simulink model "ZEH_PV_grid"  (R2020a)
settings: Solver=VariableStepAuto  StartTime=0.0  StopTime=24*60*60  RelTol=1e-3
InitFcn:
  | SENSE2_dat
values from neighbouring files (symbols this model uses):
  apv = [72 76 288 252 0 0 40 360 460 168 84]  *1E2    [ZEH_dat_summer.m]    (also in ZEH_dat_winter.m)
  cab = [0.206 0.29 0.36 285 335 ... (first row only)    [ZEH_dat_summer.m]    (also in ZEH_dat_winter.m)
  cons = [0.64,0.60,0.58,0.56,0.56,0.58,0.64,0.76,0.87,0.95,0.99,1.00,0.99,1.00,1.00,0.97,0.96,0.96,0.93,0.92,0.92,0.93,0.87,0.72]    [ZEH_dat_summer.m]    (also in ZEH_dat_winter.m = [0.67,0.63,0.60,0.59,0.59,0.60,0.74,0.86,0.85,0.96,0.96,0.95)
  inic = 0.00095    [ZEH_dat_summer.m]    (also in ZEH_dat_winter.m)
  irr = [0,0,0,0,0,0,0,0,0,0,0,0,0,0,0,0,0,0,0,0,0,0,0,0,0,0,0,0,0,0,0,0,0,0,0,0,0,0,0,0,0,0,0,0,0,0,0,0,0,0,0,0,0,0,0,0,0,0,0,0,0,0,0,0,0,0,0,0,0,0,0,0,0,0,0,0,0,0,0,0,0,0,0,0,0,0,0,0,0,0,0,0,0,0,0,0,0,0,0,0,0,0,0,0,0,0,0,0,0,0,0,0,0,0,0,0,0,0,0,0,0,0,0,0,0,0,0,0,0,0,0,0,0,0,0,0,0,0,0,0,0,0,0,0,0,0,0,0,0,0,0,0,0,0,0,0,0,0,0,0,0,0,0,0,0,0,0,0,0,0,0,0,0,0,0,0,0,0,0,0,0,0,0,0,0,0,0,0,0,0,0,0,0,0,0,0,0,0,0,0 ...(+12851 chars)    [ZEH_dat_summer.m]    (also in ZEH_dat_winter.m = zeros(1,length(irr)))
  lp = 0.002    [ZEH_dat_summer.m]    (also in ZEH_dat_winter.m)
  SL = [7.57 8.06 30.73 53.01 133.26 219.22 4.00 37.53 48.38 17.80 9.04]*1E-3    [ZEH_dat_summer.m]    (also in ZEH_dat_winter.m)
  time = [1,1.01666666666667,1.03333333333333,1.05000000000000,1.06666666666667,1.08333333333333,1.10000000000000,1.11666666666667,1.13333333333333,1.15000000000000,1.16666666666667,1.18333333333333,1.20000000000000,1.21666666666667,1.23333333333333,1.25000000000000,1.26666666666667,1.28333333333333,1.30000000000000,1.31666666666667,1.33333333333333,1.35000000000000,1.36666666666667,1.38333333333333,1.4000 ...(+22733 chars)    [ZEH_dat_summer.m]    (also in ZEH_dat_winter.m)
  to = 0.1    [ZEH_dat_summer.m]    (also in ZEH_dat_winter.m)
undefined symbols (not defined in the file or in its folder): A, B, C, D1, Dd, Delta, j
libraries: powerlib x166, simulink_extras x12, powerlib_meascontrol x11, simulink x2, factslib x2
(part 1 of 5)
settings Model: Creator=nitbh  LastModifiedBy=nitbh

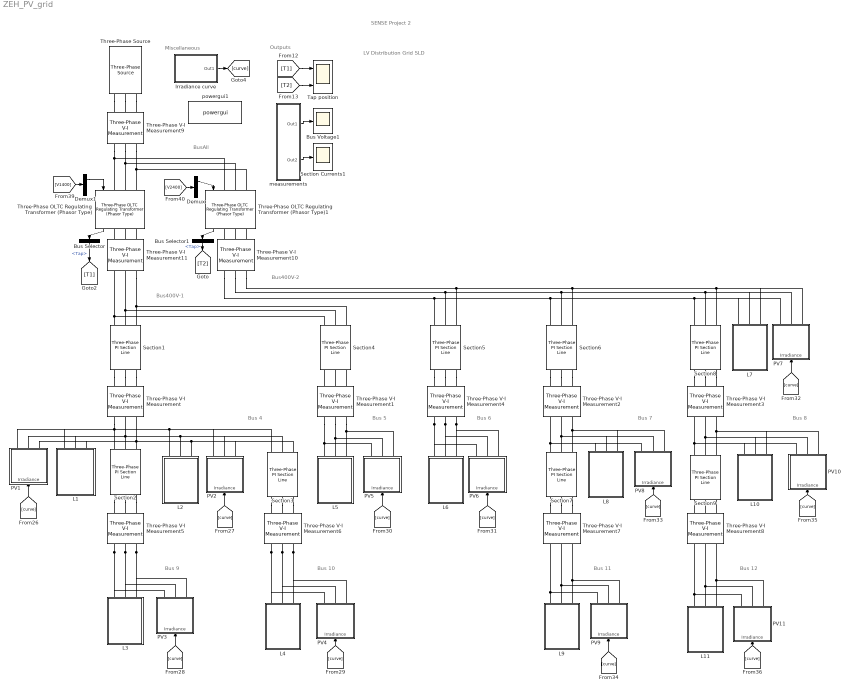
== system ZEH_PV_grid ==
  note: SENSE Project 2
  note: LV Distribution Grid SLD
  note: Outputs
  note: Miscellaneous
  note: Bus 4
  note: Bus 5
  note: Bus 9
  note: Bus 10
  note: Bus 11
  note: Bus 6
  note: Bus 7
  note: Bus 8
  note: Bus 12
  note: Bus400V-1
  note: Bus400V-2
  note: BusAll
  " Irradiance curve" : Subsystem
  Bus Selector : BusSelector  OutputSignals=Tap
  Bus Selector1 : BusSelector  OutputSignals=Tap
  Bus Voltage1 : Scope
  Demux : Demux  Outputs=3
  Demux1 : Demux  Outputs=3
  L1 : Subsystem  mask{nomPower=SL(1), PF=0.95, timestep=60, datas=cons}
      mask prompts: nomPower "Nominal Power (MW)"; PF "Power factor"; timestep "Timestep (minutes)"; datas "Consumption datas"
      mask DialogControl DescGroupVar Prompt: Load profile
      mask DialogControl DescTextVar Prompt: The load profile allows you to fix a nominal power and and a power factor. It is also needed to specify the timestep used for the consumption datas. Finally, a vector expresses the consumption profile. It has to be expressed in per unit. It is imperative that the length of the vector fits with the timestep used.
      mask Display: image(imread('Residential.jpg'))
  L10 : Subsystem  mask{nomPower=SL(10), PF=0.95, timestep=60, datas=cons}
      mask prompts: nomPower "Nominal Power (MW)"; PF "Power factor"; timestep "Timestep (minutes)"; datas "Consumption datas"
      mask DialogControl DescGroupVar Prompt: Load profile
      mask DialogControl DescTextVar Prompt: The load profile allows you to fix a nominal power and and a power factor. It is also needed to specify the timestep used for the consumption datas. Finally, a vector expresses the consumption profile. It has to be expressed in per unit. It is imperative that the length of the vector fits with the timestep used.
      mask Display: image(imread('Residential.jpg'))
  L11 : Subsystem  mask{nomPower=SL(11), PF=0.95, timestep=60, datas=cons}
      mask prompts: nomPower "Nominal Power (MW)"; PF "Power factor"; timestep "Timestep (minutes)"; datas "Consumption datas"
      mask DialogControl DescGroupVar Prompt: Load profile
      mask DialogControl DescTextVar Prompt: The load profile allows you to fix a nominal power and and a power factor. It is also needed to specify the timestep used for the consumption datas. Finally, a vector expresses the consumption profile. It has to be expressed in per unit. It is imperative that the length of the vector fits with the timestep used.
      mask Display: image(imread('Residential.jpg'))
  L2 : Subsystem  mask{nomPower=SL(2), PF=0.95, timestep=60, datas=cons}
      mask prompts: nomPower "Nominal Power (MW)"; PF "Power factor"; timestep "Timestep (minutes)"; datas "Consumption datas"
      mask DialogControl DescGroupVar Prompt: Load profile
      mask DialogControl DescTextVar Prompt: The load profile allows you to fix a nominal power and and a power factor. It is also needed to specify the timestep used for the consumption datas. Finally, a vector expresses the consumption profile. It has to be expressed in per unit. It is imperative that the length of the vector fits with the timestep used.
      mask Display: image(imread('Residential.jpg'))
  L3 : Subsystem  mask{nomPower=SL(3), PF=0.95, timestep=60, datas=cons}
      mask prompts: nomPower "Nominal Power (MW)"; PF "Power factor"; timestep "Timestep (minutes)"; datas "Consumption datas"
      mask DialogControl DescGroupVar Prompt: Load profile
      mask DialogControl DescTextVar Prompt: The load profile allows you to fix a nominal power and and a power factor. It is also needed to specify the timestep used for the consumption datas. Finally, a vector expresses the consumption profile. It has to be expressed in per unit. It is imperative that the length of the vector fits with the timestep used.
      mask Display: image(imread('Residential.jpg'))
  L4 : Subsystem  mask{nomPower=SL(4), PF=0.95, timestep=60, datas=cons}
      mask prompts: nomPower "Nominal Power (MW)"; PF "Power factor"; timestep "Timestep (minutes)"; datas "Consumption datas"
      mask DialogControl DescGroupVar Prompt: Load profile
      mask DialogControl DescTextVar Prompt: The load profile allows you to fix a nominal power and and a power factor. It is also needed to specify the timestep used for the consumption datas. Finally, a vector expresses the consumption profile. It has to be expressed in per unit. It is imperative that the length of the vector fits with the timestep used.
      mask Display: image(imread('Residential.jpg'))
  L5 : Subsystem  mask{nomPower=SL(5), PF=0.95, timestep=60, datas=cons}
      mask prompts: nomPower "Nominal Power (MW)"; PF "Power factor"; timestep "Timestep (minutes)"; datas "Consumption datas"
      mask DialogControl DescGroupVar Prompt: Load profile
      mask DialogControl DescTextVar Prompt: The load profile allows you to fix a nominal power and and a power factor. It is also needed to specify the timestep used for the consumption datas. Finally, a vector expresses the consumption profile. It has to be expressed in per unit. It is imperative that the length of the vector fits with the timestep used.
      mask Display: image(imread('Residential.jpg'))
  L6 : Subsystem  mask{nomPower=SL(6), PF=0.95, timestep=60, datas=cons}
      mask prompts: nomPower "Nominal Power (MW)"; PF "Power factor"; timestep "Timestep (minutes)"; datas "Consumption datas"
      mask DialogControl DescGroupVar Prompt: Load profile
      mask DialogControl DescTextVar Prompt: The load profile allows you to fix a nominal power and and a power factor. It is also needed to specify the timestep used for the consumption datas. Finally, a vector expresses the consumption profile. It has to be expressed in per unit. It is imperative that the length of the vector fits with the timestep used.
      mask Display: image(imread('Residential.jpg'))
  L7 : Subsystem  mask{nomPower=SL(7), PF=0.95, timestep=60, datas=cons}
      mask prompts: nomPower "Nominal Power (MW)"; PF "Power factor"; timestep "Timestep (minutes)"; datas "Consumption datas"
      mask DialogControl DescGroupVar Prompt: Load profile
      mask DialogControl DescTextVar Prompt: The load profile allows you to fix a nominal power and and a power factor. It is also needed to specify the timestep used for the consumption datas. Finally, a vector expresses the consumption profile. It has to be expressed in per unit. It is imperative that the length of the vector fits with the timestep used.
      mask Display: image(imread('Residential.jpg'))
  L8 : Subsystem  mask{nomPower=SL(8), PF=0.95, timestep=60, datas=cons}
      mask prompts: nomPower "Nominal Power (MW)"; PF "Power factor"; timestep "Timestep (minutes)"; datas "Consumption datas"
      mask DialogControl DescGroupVar Prompt: Load profile
      mask DialogControl DescTextVar Prompt: The load profile allows you to fix a nominal power and and a power factor. It is also needed to specify the timestep used for the consumption datas. Finally, a vector expresses the consumption profile. It has to be expressed in per unit. It is imperative that the length of the vector fits with the timestep used.
      mask Display: image(imread('Residential.jpg'))
  L9 : Subsystem  mask{nomPower=SL(9), PF=0.95, timestep=60, datas=cons}
      mask prompts: nomPower "Nominal Power (MW)"; PF "Power factor"; timestep "Timestep (minutes)"; datas "Consumption datas"
      mask DialogControl DescGroupVar Prompt: Load profile
      mask DialogControl DescTextVar Prompt: The load profile allows you to fix a nominal power and and a power factor. It is also needed to specify the timestep used for the consumption datas. Finally, a vector expresses the consumption profile. It has to be expressed in per unit. It is imperative that the length of the vector fits with the timestep used.
      mask Display: image(imread('Residential.jpg'))
  PV1 : Subsystem  mask{eff=10, area=apv(1)}
      mask prompts: eff "Efficiency (%)"; area "Area (m^2)"
      mask help: The product of the effeciency, the area covered by the Pv farm and the irradiance in w/m2 will give you the power generate by the PV farm.
      mask DialogControl DescGroupVar Prompt: PV farm
      mask DialogControl DescTextVar Prompt: The product of the efficiency, the area covered by the PV farm and the irradiance in W/m2 will give you the power generated by the PV farm.
      mask Display: image(imread('panel.jpg'))
  PV10 : Subsystem  mask{eff=10, area=apv(10)}
      mask prompts: eff "Efficiency (%)"; area "Area (m^2)"
      mask help: The product of the effeciency, the area covered by the Pv farm and the irradiance in w/m2 will give you the power generate by the PV farm.
      mask DialogControl DescGroupVar Prompt: PV farm
      mask DialogControl DescTextVar Prompt: The product of the efficiency, the area covered by the PV farm and the irradiance in W/m2 will give you the power generated by the PV farm.
      mask Display: image(imread('panel.jpg'))
  PV11 : Subsystem  mask{eff=10, area=apv(11)}
      mask prompts: eff "Efficiency (%)"; area "Area (m^2)"
      mask help: The product of the effeciency, the area covered by the Pv farm and the irradiance in w/m2 will give you the power generate by the PV farm.
      mask DialogControl DescGroupVar Prompt: PV farm
      mask DialogControl DescTextVar Prompt: The product of the efficiency, the area covered by the PV farm and the irradiance in W/m2 will give you the power generated by the PV farm.
      mask Display: image(imread('panel.jpg'))
  PV2 : Subsystem  mask{eff=10, area=apv(2)}
      mask prompts: eff "Efficiency (%)"; area "Area (m^2)"
      mask help: The product of the effeciency, the area covered by the Pv farm and the irradiance in w/m2 will give you the power generate by the PV farm.
      mask DialogControl DescGroupVar Prompt: PV farm
      mask DialogControl DescTextVar Prompt: The product of the efficiency, the area covered by the PV farm and the irradiance in W/m2 will give you the power generated by the PV farm.
      mask Display: image(imread('panel.jpg'))
  PV3 : Subsystem  mask{eff=10, area=apv(3)}
      mask prompts: eff "Efficiency (%)"; area "Area (m^2)"
      mask help: The product of the effeciency, the area covered by the Pv farm and the irradiance in w/m2 will give you the power generate by the PV farm.
      mask DialogControl DescGroupVar Prompt: PV farm
      mask DialogControl DescTextVar Prompt: The product of the efficiency, the area covered by the PV farm and the irradiance in W/m2 will give you the power generated by the PV farm.
      mask Display: image(imread('panel.jpg'))
  PV4 : Subsystem  mask{eff=10, area=apv(4)}
      mask prompts: eff "Efficiency (%)"; area "Area (m^2)"
      mask help: The product of the effeciency, the area covered by the Pv farm and the irradiance in w/m2 will give you the power generate by the PV farm.
      mask DialogControl DescGroupVar Prompt: PV farm
      mask DialogControl DescTextVar Prompt: The product of the efficiency, the area covered by the PV farm and the irradiance in W/m2 will give you the power generated by the PV farm.
      mask Display: image(imread('panel.jpg'))
  PV5 : Subsystem  mask{eff=10, area=apv(5)}
      mask prompts: eff "Efficiency (%)"; area "Area (m^2)"
      mask help: The product of the effeciency, the area covered by the Pv farm and the irradiance in w/m2 will give you the power generate by the PV farm.
      mask DialogControl DescGroupVar Prompt: PV farm
      mask DialogControl DescTextVar Prompt: The product of the efficiency, the area covered by the PV farm and the irradiance in W/m2 will give you the power generated by the PV farm.
      mask Display: image(imread('panel.jpg'))
  PV6 : Subsystem  mask{eff=10, area=apv(6)}
      mask prompts: eff "Efficiency (%)"; area "Area (m^2)"
      mask help: The product of the effeciency, the area covered by the Pv farm and the irradiance in w/m2 will give you the power generate by the PV farm.
      mask DialogControl DescGroupVar Prompt: PV farm
      mask DialogControl DescTextVar Prompt: The product of the efficiency, the area covered by the PV farm and the irradiance in W/m2 will give you the power generated by the PV farm.
      mask Display: image(imread('panel.jpg'))
  PV7 : Subsystem  mask{eff=10, area=apv(7)}
      mask prompts: eff "Efficiency (%)"; area "Area (m^2)"
      mask help: The product of the effeciency, the area covered by the Pv farm and the irradiance in w/m2 will give you the power generate by the PV farm.
      mask DialogControl DescGroupVar Prompt: PV farm
      mask DialogControl DescTextVar Prompt: The product of the efficiency, the area covered by the PV farm and the irradiance in W/m2 will give you the power generated by the PV farm.
      mask Display: image(imread('panel.jpg'))
  PV8 : Subsystem  mask{eff=10, area=apv(8)}
      mask prompts: eff "Efficiency (%)"; area "Area (m^2)"
      mask help: The product of the effeciency, the area covered by the Pv farm and the irradiance in w/m2 will give you the power generate by the PV farm.
      mask DialogControl DescGroupVar Prompt: PV farm
      mask DialogControl DescTextVar Prompt: The product of the efficiency, the area covered by the PV farm and the irradiance in W/m2 will give you the power generated by the PV farm.
      mask Display: image(imread('panel.jpg'))
  PV9 : Subsystem  mask{eff=10, area=apv(9)}
      mask prompts: eff "Efficiency (%)"; area "Area (m^2)"
      mask help: The product of the effeciency, the area covered by the Pv farm and the irradiance in w/m2 will give you the power generate by the PV farm.
      mask DialogControl DescGroupVar Prompt: PV farm
      mask DialogControl DescTextVar Prompt: The product of the efficiency, the area covered by the PV farm and the irradiance in W/m2 will give you the power generated by the PV farm.
      mask Display: image(imread('panel.jpg'))
  Section Currents1 : Scope
  Section1 : powerlib/Elements/Three-Phase PI Section Line  LConnTagsString=a|b|c  RConnTagsString=A|B|C  Length=0.02  Frequency=50  Resistances=[ cab(1,1) 0.3864]  Inductances="[ cab(1,2)  4.1264e-3]"  Capacitances=[cab(1,3) 7.751e-9]
  Section2 : powerlib/Elements/Three-Phase PI Section Line  LConnTagsString=a|b|c  RConnTagsString=A|B|C  Length=0.1  Frequency=50  Resistances=[ cab(2,1) 0.3864]  Inductances="[ cab(2,2)  4.1264e-3]"  Capacitances=[ cab(2,3) 7.751e-9]
  Section3 : powerlib/Elements/Three-Phase PI Section Line  LConnTagsString=a|b|c  RConnTagsString=A|B|C  Length=0.2  Frequency=50  Resistances=[ cab(3,1) 0.3864]  Inductances="[ cab(3,2)  4.1264e-3]"  Capacitances=[cab(3,3) 7.751e-9]
  Section4 : powerlib/Elements/Three-Phase PI Section Line  LConnTagsString=a|b|c  RConnTagsString=A|B|C  Length=0.13  Frequency=50  Resistances=[ cab(4,1) 0.3864]  Inductances="[ cab(4,2)  4.1264e-3]"  Capacitances=[cab(4,3) 7.751e-9]
  Section5 : powerlib/Elements/Three-Phase PI Section Line  LConnTagsString=a|b|c  RConnTagsString=A|B|C  Length=0.13  Frequency=50  Resistances=[ cab(5,1) 0.3864]  Inductances="[ cab(5,2)  4.1264e-3]"  Capacitances=[cab(5,3) 7.751e-9]
  Section6 : powerlib/Elements/Three-Phase PI Section Line  LConnTagsString=a|b|c  RConnTagsString=A|B|C  Length=0.2  Frequency=50  Resistances=[ cab(6,1) 0.3864]  Inductances="[ cab(6,2)  4.1264e-3]"  Capacitances=[cab(2,3) 7.751e-9]
  Section7 : powerlib/Elements/Three-Phase PI Section Line  LConnTagsString=a|b|c  RConnTagsString=A|B|C  Length=0.07  Frequency=50  Resistances=[ cab(7,1) 0.3864]  Inductances="[cab(7,2)  4.1264e-3]"  Capacitances=[cab(7,3) 7.751e-9]
  Section8 : powerlib/Elements/Three-Phase PI Section Line  LConnTagsString=a|b|c  RConnTagsString=A|B|C  Length=0.1  Frequency=50  Resistances=[ cab(8,1) 0.3864]  Inductances="[ cab(8,2)  4.1264e-3]"  Capacitances=[cab(8,3) 7.751e-9]
  Section9 : powerlib/Elements/Three-Phase PI Section Line  LConnTagsString=a|b|c  RConnTagsString=A|B|C  Length=0.1  Frequency=50  Resistances=[ cab(9,1) 0.3864]  Inductances="[ cab(9,2)  4.1264e-3]"  Capacitances=[cab(9,3) 7.751e-9]
  Tap position : Scope  NumInputPorts=2
  Three-Phase V-I Measurement : powerlib/Measurements/Three-Phase V-I Measurement  VoltageMeasurement=phase-to-phase  SetLabelV=on  LabelV=VS1  Vpu=off  VpuLL=on  CurrentMeasurement=yes  SetLabelI=on  LabelI=IS1  Ipu=on  Pbase=800e3  Vbase=420  OutputType=Magnitude  PhasorSimulation=on  PSBequivalent=0
  Three-Phase V-I Measurement1 : powerlib/Measurements/Three-Phase V-I Measurement  VoltageMeasurement=phase-to-phase  SetLabelV=on  LabelV=VS4  Vpu=off  VpuLL=on  CurrentMeasurement=yes  SetLabelI=on  LabelI=IS4  Ipu=on  Pbase=800e3  Vbase=420  OutputType=Magnitude  PhasorSimulation=on  PSBequivalent=0
  Three-Phase V-I Measurement10 : powerlib/Measurements/Three-Phase V-I Measurement  VoltageMeasurement=phase-to-phase  SetLabelV=on  LabelV=V2400  Vpu=off  VpuLL=on  CurrentMeasurement=yes  SetLabelI=on  LabelI=I2400  Ipu=on  Pbase=800e3  Vbase=420  OutputType=Magnitude  PhasorSimulation=on  PSBequivalent=0
  Three-Phase V-I Measurement11 : powerlib/Measurements/Three-Phase V-I Measurement  VoltageMeasurement=phase-to-phase  SetLabelV=on  LabelV=V1400  Vpu=off  VpuLL=on  CurrentMeasurement=yes  SetLabelI=on  LabelI=I1400  Ipu=on  Pbase=800e3  Vbase=420  OutputType=Magnitude  PhasorSimulation=on  PSBequivalent=0
  Three-Phase V-I Measurement2 : powerlib/Measurements/Three-Phase V-I Measurement  VoltageMeasurement=phase-to-phase  SetLabelV=on  LabelV=VS6  Vpu=off  VpuLL=on  CurrentMeasurement=yes  SetLabelI=on  LabelI=IS6  Ipu=on  Pbase=800e3  Vbase=420  OutputType=Magnitude  PhasorSimulation=on  PSBequivalent=0
  Three-Phase V-I Measurement3 : powerlib/Measurements/Three-Phase V-I Measurement  VoltageMeasurement=phase-to-phase  SetLabelV=on  LabelV=VS8  Vpu=off  VpuLL=on  CurrentMeasurement=yes  SetLabelI=on  LabelI=IS8  Ipu=on  Pbase=800e3  Vbase=420  OutputType=Magnitude  PhasorSimulation=on  PSBequivalent=0
  Three-Phase V-I Measurement4 : powerlib/Measurements/Three-Phase V-I Measurement  VoltageMeasurement=phase-to-phase  SetLabelV=on  LabelV=VS5  Vpu=off  VpuLL=on  CurrentMeasurement=yes  SetLabelI=on  LabelI=IS5  Ipu=on  Pbase=800e3  Vbase=420  OutputType=Magnitude  PhasorSimulation=on  PSBequivalent=0
  Three-Phase V-I Measurement5 : powerlib/Measurements/Three-Phase V-I Measurement  VoltageMeasurement=phase-to-phase  SetLabelV=on  LabelV=VS2  Vpu=off  VpuLL=on  CurrentMeasurement=yes  SetLabelI=on  LabelI=IS2  Ipu=on  Pbase=800e3  Vbase=420  OutputType=Magnitude  PhasorSimulation=on  PSBequivalent=0
  Three-Phase V-I Measurement6 : powerlib/Measurements/Three-Phase V-I Measurement  VoltageMeasurement=phase-to-phase  SetLabelV=on  LabelV=VS3  Vpu=off  VpuLL=on  CurrentMeasurement=yes  SetLabelI=on  LabelI=IS3  Ipu=on  Pbase=800e3  Vbase=420  OutputType=Magnitude  PhasorSimulation=on  PSBequivalent=0
  Three-Phase V-I Measurement7 : powerlib/Measurements/Three-Phase V-I Measurement  VoltageMeasurement=phase-to-phase  SetLabelV=on  LabelV=VS7  Vpu=off  VpuLL=on  CurrentMeasurement=yes  SetLabelI=on  LabelI=IS7  Ipu=on  Pbase=800e3  Vbase=420  OutputType=Magnitude  PhasorSimulation=on  PSBequivalent=0
  Three-Phase V-I Measurement8 : powerlib/Measurements/Three-Phase V-I Measurement  VoltageMeasurement=phase-to-phase  SetLabelV=on  LabelV=VS9  Vpu=off  VpuLL=on  CurrentMeasurement=yes  SetLabelI=on  LabelI=IS9  Ipu=on  Pbase=800e3  Vbase=420  OutputType=Magnitude  PhasorSimulation=on  PSBequivalent=0
  Three-Phase V-I Measurement9 : powerlib/Measurements/Three-Phase V-I Measurement  VoltageMeasurement=phase-to-phase  SetLabelV=on  LabelV=Vall  Vpu=off  VpuLL=on  CurrentMeasurement=yes  SetLabelI=on  LabelI=Iall  Ipu=on  Pbase=800e3  Vbase=11e3  OutputType=Magnitude  PhasorSimulation=on  PSBequivalent=0
  Three-Phase OLTC Regulating Transformer (Phasor Type) : factslib/Transformers/Three-Phase OLTC Regulating Transformer (Phasor Type)  Winding1Connection=Delta (D1)  Winding2Connection=Yg  PnomFnom="[0.8e6,  50]"  Winding1=[11e3, 0.00829, 0.04829 ]  Winding2="[420,  0.00829, 0.04829 ]"  Iw2_init=[0.7568, -45]  RmXm=[300, 300]  TapOnWinding=Winding 1  WindingTap=[ 0.003, 0.09]  dU=0.01875  TapMinMax=[ -8, +8]  InitialTap=-4  TapSelectionTime=0.001  ExternalControl=off  RegulatorOn=on  Regulator="[1.04,  0.0375, 1]"
      settings: SourceProductBaseCode=PS
  Three-Phase OLTC Regulating Transformer (Phasor Type)1 : factslib/Transformers/Three-Phase OLTC Regulating Transformer (Phasor Type)  Winding1Connection=Delta (D1)  Winding2Connection=Yg  PnomFnom="[0.8e6,  50]"  Winding1=[11e3, 0.00829, 0.04829 ]  Winding2="[420,  0.00829, 0.04829 ]"  Iw2_init=[0.7568, -45]  RmXm=[300, 300]  TapOnWinding=Winding 1  WindingTap=[ 0.003, 0.09]  dU=0.01875  TapMinMax=[ -8, +8]  InitialTap=-4  TapSelectionTime=0.001  ExternalControl=off  RegulatorOn=on  Regulator="[1.04,  0.0375, 1]"
      settings: SourceProductBaseCode=PS
  Three-Phase Source : powerlib/Electrical Sources/Three-Phase Source  InternalConnection=Yg  VoltagePhases=off  Voltage=11e3  PhaseAngle=0  Voltage_phases=[25e3 25e3 25e3]/sqrt(3)  PhaseAngles_phases=[0 -120 +120]  Frequency=50  NonIdealSource=off  SpecifyImpedance=off  Resistance=0.8929  Inductance=16.58e-3  ShortCircuitLevel=100e6  BaseVoltage=11e3  XRratio=7  BusType=swing  Pref=10e3  Qref=0  Prefabc=[10e3, 10e3, 10e3]  Qrefabc=[0, 0, 0]  Qmin=-inf  Qmax=inf
  measurements : Subsystem
  powergui1 : powerlib/powergui  Priority=1  SimulationMode=Phasor  SampleTime=50e-6  frequency=50  Iterations=50  frequencyindice=50  Pbase=10e6  ErrMax=0.0001  UnitsV=kV  UnitsW=MW  buscounter=0  FunctionMessages=off  echomessages=off  EnableUseOfTLC=off  CurrentSourceSwitches=off  DisableSnubberDevices=off  DisableRonSwitches=off  DisableVfSwitches=off  DisplayEquations=off  AutomaticDiscreteSolvers=off  SolverType=Tustin  Interpol=off  ExternalGateDelay=off  methode=off  Ts=100  x0status=blocks  SPID=off  SwTol=0  HookPort=off  NonlinearTolerance=0  nMaxIteration=15  ContinueOnMaxIteration=off  RestoreLinks=warning  ResistiveCurrentMeasurement=off  Frange=[0:2:500]  Ylog=off  Xlog=on  ShowGrid=off  save=off  variable=ZData  structure=0  ZoomFFT=off  StartTime=0.0  cycles=1  DisplayStyle=1  fundamental=60  FreqAxis=off  MaxFrequency=1000  frequencyindicesteady=1  RmsSteady=1  display=off
  wires:
  [curve] -> PV1/1(Irradiance)
  [curve] -> PV2/1(Irradiance)
  [curve] -> PV3/1(Irradiance)
  [curve] -> PV4/1(Irradiance)
  [curve] -> PV5/1(Irradiance)
  [curve] -> PV6/1(Irradiance)
  [curve] -> PV7/1(Irradiance)
  [curve] -> PV8/1(Irradiance)
  [curve] -> PV9/1(Irradiance)
  [curve] -> PV10/1(Irradiance)
  [curve] -> PV11/1(Irradiance)
  Demux1/1 -> Three-Phase OLTC Regulating Transformer (Phasor Type)/1
  Demux/1 -> Three-Phase OLTC Regulating Transformer (Phasor Type)1/1
  [V2400] -> Demux/1
  [V1400] -> Demux1/1
  Bus Selector/1 -> [T1]  "<Tap>"
  Three-Phase OLTC Regulating Transformer (Phasor Type)/1 -> Bus Selector/1
  Bus Selector1/1 -> [T2]  "<Tap>"
  Three-Phase OLTC Regulating Transformer (Phasor Type)1/1 -> Bus Selector1/1
  measurements/1(Out1) -> Bus Voltage1/1
  measurements/2(Out2) -> Section Currents1/1
  [T2] -> Tap position/2
  [T1] -> Tap position/1
  " Irradiance curve"/1(Out1) -> [curve]
  connections:
  Three-Phase V-I Measurement9/RConn1 -- Three-Phase OLTC Regulating Transformer (Phasor Type)/LConn1 -- Three-Phase OLTC Regulating Transformer (Phasor Type)1/LConn1
  Three-Phase V-I Measurement9/RConn2 -- Three-Phase OLTC Regulating Transformer (Phasor Type)/LConn2 -- Three-Phase OLTC Regulating Transformer (Phasor Type)1/LConn2
  Three-Phase V-I Measurement9/RConn3 -- Three-Phase OLTC Regulating Transformer (Phasor Type)/LConn3 -- Three-Phase OLTC Regulating Transformer (Phasor Type)1/LConn3
  Three-Phase Source/RConn1 -- Three-Phase V-I Measurement9/LConn1
  Three-Phase Source/RConn2 -- Three-Phase V-I Measurement9/LConn2
  Three-Phase Source/RConn3 -- Three-Phase V-I Measurement9/LConn3
  Section1/RConn1 -- Three-Phase V-I Measurement/LConn1
  Section1/RConn2 -- Three-Phase V-I Measurement/LConn2
  Section1/RConn3 -- Three-Phase V-I Measurement/LConn3
  Section5/LConn1 -- Three-Phase V-I Measurement10/RConn1 -- L7/LConn1 -- PV7/RConn1 -- Section8/LConn1 -- Section6/LConn1
  Section5/LConn2 -- Three-Phase V-I Measurement10/RConn2 -- L7/LConn2 -- PV7/RConn2 -- Section8/LConn2 -- Section6/LConn2
  Section5/LConn3 -- Three-Phase V-I Measurement10/RConn3 -- L7/LConn3 -- PV7/RConn3 -- Section8/LConn3 -- Section6/LConn3
  Three-Phase V-I Measurement/RConn1 -- PV1/RConn1 -- L1/LConn1 -- Section3/LConn1 -- PV2/RConn1 -- L2/LConn1 -- Section2/LConn1
  Section2/LConn2 -- L1/LConn2 -- PV1/RConn2 -- Section3/LConn2 -- PV2/RConn2 -- L2/LConn2 -- Three-Phase V-I Measurement/RConn2
  Section2/LConn3 -- PV1/RConn3 -- L1/LConn3 -- Section3/LConn3 -- PV2/RConn3 -- L2/LConn3 -- Three-Phase V-I Measurement/RConn3
  Section2/RConn1 -- Three-Phase V-I Measurement5/LConn1
  Section2/RConn2 -- Three-Phase V-I Measurement5/LConn2
  Section2/RConn3 -- Three-Phase V-I Measurement5/LConn3
  Three-Phase V-I Measurement5/RConn1 -- L3/LConn1 -- PV3/RConn1
  Three-Phase V-I Measurement5/RConn2 -- L3/LConn2 -- PV3/RConn2
  Three-Phase V-I Measurement5/RConn3 -- L3/LConn3 -- PV3/RConn3
  Three-Phase V-I Measurement6/RConn1 -- L4/LConn1 -- PV4/RConn1
  Three-Phase V-I Measurement6/RConn2 -- L4/LConn2 -- PV4/RConn2
  Three-Phase V-I Measurement6/RConn3 -- L4/LConn3 -- PV4/RConn3
  Section3/RConn1 -- Three-Phase V-I Measurement6/LConn1
  Section3/RConn2 -- Three-Phase V-I Measurement6/LConn2
  Section3/RConn3 -- Three-Phase V-I Measurement6/LConn3
  Three-Phase V-I Measurement1/RConn1 -- L5/LConn1 -- PV5/RConn1
  Three-Phase V-I Measurement1/RConn2 -- L5/LConn2 -- PV5/RConn2
  Three-Phase V-I Measurement1/RConn3 -- L5/LConn3 -- PV5/RConn3
  Three-Phase V-I Measurement1/LConn1 -- Section4/RConn1
  Three-Phase V-I Measurement1/LConn2 -- Section4/RConn2
  Three-Phase V-I Measurement1/LConn3 -- Section4/RConn3
  Three-Phase V-I Measurement4/RConn1 -- L6/LConn1 -- PV6/RConn1
  Three-Phase V-I Measurement4/RConn2 -- L6/LConn2 -- PV6/RConn2
  Three-Phase V-I Measurement4/RConn3 -- L6/LConn3 -- PV6/RConn3
  Section5/RConn1 -- Three-Phase V-I Measurement4/LConn1
  Section5/RConn2 -- Three-Phase V-I Measurement4/LConn2
  Section5/RConn3 -- Three-Phase V-I Measurement4/LConn3
  Section6/RConn1 -- Three-Phase V-I Measurement2/LConn1
  Section6/RConn2 -- Three-Phase V-I Measurement2/LConn2
  Section6/RConn3 -- Three-Phase V-I Measurement2/LConn3
  Section8/RConn1 -- Three-Phase V-I Measurement3/LConn1
  Section8/RConn2 -- Three-Phase V-I Measurement3/LConn2
  Section8/RConn3 -- Three-Phase V-I Measurement3/LConn3
  L9/LConn1 -- Three-Phase V-I Measurement7/RConn1 -- PV9/RConn1
  L9/LConn2 -- Three-Phase V-I Measurement7/RConn2 -- PV9/RConn2
  L9/LConn3 -- Three-Phase V-I Measurement7/RConn3 -- PV9/RConn3
  Section7/RConn1 -- Three-Phase V-I Measurement7/LConn1
  Section7/RConn2 -- Three-Phase V-I Measurement7/LConn2
  Section7/RConn3 -- Three-Phase V-I Measurement7/LConn3
  Section7/LConn1 -- L8/LConn1 -- PV8/RConn1 -- Three-Phase V-I Measurement2/RConn1
  Section7/LConn2 -- L8/LConn2 -- PV8/RConn2 -- Three-Phase V-I Measurement2/RConn2
  Section7/LConn3 -- L8/LConn3 -- PV8/RConn3 -- Three-Phase V-I Measurement2/RConn3
  Section9/LConn1 -- Three-Phase V-I Measurement3/RConn1 -- L10/LConn1 -- PV10/RConn1
  Section9/LConn2 -- L10/LConn2 -- PV10/RConn2 -- Three-Phase V-I Measurement3/RConn2
  Section9/LConn3 -- L10/LConn3 -- PV10/RConn3 -- Three-Phase V-I Measurement3/RConn3
  Three-Phase V-I Measurement8/LConn1 -- Section9/RConn1
  Three-Phase V-I Measurement8/LConn2 -- Section9/RConn2
  Three-Phase V-I Measurement8/LConn3 -- Section9/RConn3
  L11/LConn1 -- Three-Phase V-I Measurement8/RConn1 -- PV11/RConn1
  L11/LConn2 -- Three-Phase V-I Measurement8/RConn2 -- PV11/RConn2
  L11/LConn3 -- PV11/RConn3 -- Three-Phase V-I Measurement8/RConn3
  Section1/LConn3 -- Section4/LConn3 -- Three-Phase V-I Measurement11/RConn3
  Section4/LConn1 -- Three-Phase V-I Measurement11/RConn1 -- Section1/LConn1
  Section4/LConn2 -- Three-Phase V-I Measurement11/RConn2 -- Section1/LConn2
  Three-Phase V-I Measurement10/LConn1 -- Three-Phase OLTC Regulating Transformer (Phasor Type)1/RConn1
  Three-Phase V-I Measurement10/LConn2 -- Three-Phase OLTC Regulating Transformer (Phasor Type)1/RConn2
  Three-Phase V-I Measurement10/LConn3 -- Three-Phase OLTC Regulating Transformer (Phasor Type)1/RConn3
  Three-Phase V-I Measurement11/LConn1 -- Three-Phase OLTC Regulating Transformer (Phasor Type)/RConn1
  Three-Phase V-I Measurement11/LConn2 -- Three-Phase OLTC Regulating Transformer (Phasor Type)/RConn2
  Three-Phase V-I Measurement11/LConn3 -- Three-Phase OLTC Regulating Transformer (Phasor Type)/RConn3

== system ZEH_PV_grid/ Irradiance curve ==
  Irradiance : Subsystem
      mask init:
      | load power_V2G
      mask Display: plot(V2G.IRRADIANCE.time,V2G.IRRADIANCE.SUN)
  Partial Shading : Subsystem  mask(Signal Disturbance){Hour=12, Minute=0, Second=0, Duration=5*60, Factor=0.7}
      mask prompts: Duration "Duration (s):"
      mask help: Within the specified time range defined by Start and Duration parameters, output is set to 'Factor'. Outside the specified time range output is kept at 1.0.
      mask init:
      | T2=(Hour-1)*60*60;    % Hour in seconds
      | T3=(Minute-1)*60;  % Minute in seconds
      | Ton=T2+T3+(Second-1);    % Beginning of fault (s)
      | Toff=Ton+Duration; % End of fault (s)
      mask TypeOptions Hour: 0 |      1 |      2 |      3 |      4 |      5 |      6 |      7 |      8 |      9 |     10 |     11 |     12 |     13 |     14 |     15 |     16 |     17 |     18 |     19 |     20 |     21 |     22 |     23
      mask TypeOptions Minute: 0 |      1 |      2 |      3 |      4 |      5 |      6 |      7 |      8 |      9 |     10 |     11 |     12 |     13 |     14 |     15 |     16 |     17 |     18 |     19 |     20 |     21 |     22 |     23 |     24 |     25 |     26 |     27 |     28 |     29 |     30 |     31 |     32 |     33 |     34 |     35 |     36 |     37 |     38 |     39 |     40 |     41 |     42 |     43 |     44 |     45 |     46 |     47 |     48 |     49 |     50 |     51 |     52 |     53 |     54 |     55 |     56 |     57 |     58 |     59
      mask TypeOptions Second: 0 |      1 |      2 |      3 |      4 |      5 |      6 |      7 |      8 |      9 |     10 |     11 |     12 |     13 |     14 |     15 |     16 |     17 |     18 |     19 |     20 |     21 |     22 |     23 |     24 |     25 |     26 |     27 |     28 |     29 |     30 |     31 |     32 |     33 |     34 |     35 |     36 |     37 |     38 |     39 |     40 |     41 |     42 |     43 |     44 |     45 |     46 |     47 |     48 |     49 |     50 |     51 |     52 |     53 |     54 |     55 |     56 |     57 |     58 |     59
      mask DialogControl Control2 Prompt: Start:
  Product1 : Product
  Rate Limiter2 : RateLimiter  RisingSlewLimit=1e4  FallingSlewLimit=-1e4  SampleTimeMode=inherited
  Out1 : Outport
  wires:
  Rate Limiter2/1 -> Out1/1
  Product1/1 -> Rate Limiter2/1
  Partial Shading/1(Out) -> Product1/2
  Irradiance/1(" ") -> Product1/1

== system ZEH_PV_grid/L1 ==
  note: V1= 1/3(Vab -a^2*Vbc)
  note: S = 3* ( V * I') / 2
  note: Ia= I1
  note: Ib= a^2*I1
  Add : Sum  Inputs=+-
  Avoid division by zero : Subsystem
  Break Alg. Loop 1 : Subsystem
  CSb : powerlib/Electrical Sources/Controlled Current Source  Initialize=on  Source_Type=AC  Amplitude=9355.5  Phase=(2.751-2*pi/3)*180/pi  Frequency=60  Measurements=Current
  Conj1 : Math  Operator=conj  SignedPower=on  SaturateOnIntegerOverflow=on
  Csa : powerlib/Electrical Sources/Controlled Current Source  Initialize=on  Source_Type=AC  Amplitude=9355.5  Phase=2.751*180/pi  Frequency=60  Measurements=Current
  Demux : Demux  Outputs=2
  Load : Subsystem
  Product : Product  Inputs=/*  InputSameDT=on  SaturateOnIntegerOverflow=on  OutDataTypeStr=Inherit: Same as first input
  Real-Imag to Complex : RealImagToComplex
  Series RLC Branch : powerlib/Elements/Series RLC Branch  LConnTagsString=__new0  RConnTagsString=__new0  BranchType=R  Resistance=1e6  Inductance=1e-3  SetiL0=off  InitialCurrent=0  Capacitance=1e-6  Setx0=off  InitialVoltage=0  Measurements=None
  Series RLC Branch1 : powerlib/Elements/Series RLC Branch  LConnTagsString=__new0  RConnTagsString=__new0  BranchType=R  Resistance=1e6  Inductance=1e-3  SetiL0=off  InitialCurrent=0  Capacitance=1e-6  Setx0=off  InitialVoltage=0  Measurements=None
  Voltage Measurement1 : powerlib/Measurements/Voltage Measurement  PhasorSimulation=on  OutputType=Complex  PSBequivalent=0
  Voltage Measurement2 : powerlib/Measurements/Voltage Measurement  PhasorSimulation=on  OutputType=Complex  PSBequivalent=0
  a^2 : Gain  Gain=exp(-j*2*pi/3)  SaturateOnIntegerOverflow=on  OutDataTypeStr=Inherit: Same as input  ParamDataTypeStr=Inherit: Same as input
  "a^2 " : Gain  Gain=exp(-j*2*pi/3)  SaturateOnIntegerOverflow=on  OutDataTypeStr=Inherit: Same as input  ParamDataTypeStr=Inherit: Same as input
  a^3 : Gain  Gain=1/3  SaturateOnIntegerOverflow=on  OutDataTypeStr=Inherit: Same as input  ParamDataTypeStr=Inherit: Same as input
  a^4 : Gain  Gain=2/3  SaturateOnIntegerOverflow=on  OutDataTypeStr=Inherit: Same as input  ParamDataTypeStr=Inherit: Same as input
  A : PMIOPort  Tag=PMCPort  Side=Left
  B : PMIOPort  Tag=PMCPort  Port=2  Side=Left
  C : PMIOPort  Tag=PMCPort  Port=3  Side=Left
  wires:
  Voltage Measurement1/1 -> [Vab]
  Voltage Measurement2/1 -> [Vbc]
  [Ia] -> Csa/1
  [Ib] -> CSb/1
  Real-Imag to Complex/1 -> Product/2
  Product/1 -> a^4/1  "I1"
  a^2/1 -> [Ib]
  a^3/1 -> Avoid division by zero/1(I)
  Add/1 -> a^3/1
  [Vab] -> Add/1
  [Vbc] -> "a^2 "/1
  "a^2 "/1 -> Add/2
  a^4/1 -> Conj1/1
  Demux/1 -> Real-Imag to Complex/1
  Demux/2 -> Real-Imag to Complex/2
  Load/1(PQ) -> Demux/1
  Avoid division by zero/1(O) -> Product/1  "V1"
  Conj1/1 -> Break Alg. Loop 1/1(In)
  Break Alg. Loop 1/1(Out) -> [Ia], a^2/1
  connections:
  Series RLC Branch/LConn1 -- A/RConn1 -- Csa/RConn1 -- Voltage Measurement1/LConn1
  Voltage Measurement2/LConn2 -- C/RConn1 -- Series RLC Branch1/RConn1 -- Csa/LConn1 -- CSb/LConn1
  CSb/RConn1 -- Voltage Measurement2/LConn1 -- Voltage Measurement1/LConn2 -- B/RConn1 -- Series RLC Branch1/LConn1 -- Series RLC Branch/RConn1

== system ZEH_PV_grid/L10 ==
  note: Ib= a^2*I1
  note: Ia= I1
  note: S = 3* ( V * I') / 2
  note: V1= 1/3(Vab -a^2*Vbc)
  Add : Sum  Inputs=+-
  Avoid division by zero : Subsystem
  Break Alg. Loop 1 : Subsystem
  CSb : powerlib/Electrical Sources/Controlled Current Source  Initialize=on  Source_Type=AC  Amplitude=9355.5  Phase=(2.751-2*pi/3)*180/pi  Frequency=60  Measurements=Current
  Conj1 : Math  Operator=conj  SignedPower=on  SaturateOnIntegerOverflow=on
  Csa : powerlib/Electrical Sources/Controlled Current Source  Initialize=on  Source_Type=AC  Amplitude=9355.5  Phase=2.751*180/pi  Frequency=60  Measurements=Current
  Demux : Demux  Outputs=2
  Load : Subsystem
  Product : Product  Inputs=/*  InputSameDT=on  SaturateOnIntegerOverflow=on  OutDataTypeStr=Inherit: Same as first input
  Real-Imag to Complex : RealImagToComplex
  Series RLC Branch : powerlib/Elements/Series RLC Branch  LConnTagsString=__new0  RConnTagsString=__new0  BranchType=R  Resistance=1e6  Inductance=1e-3  SetiL0=off  InitialCurrent=0  Capacitance=1e-6  Setx0=off  InitialVoltage=0  Measurements=None
  Series RLC Branch1 : powerlib/Elements/Series RLC Branch  LConnTagsString=__new0  RConnTagsString=__new0  BranchType=R  Resistance=1e6  Inductance=1e-3  SetiL0=off  InitialCurrent=0  Capacitance=1e-6  Setx0=off  InitialVoltage=0  Measurements=None
  Voltage Measurement1 : powerlib/Measurements/Voltage Measurement  PhasorSimulation=on  OutputType=Complex  PSBequivalent=0
  Voltage Measurement2 : powerlib/Measurements/Voltage Measurement  PhasorSimulation=on  OutputType=Complex  PSBequivalent=0
  a^2 : Gain  Gain=exp(-j*2*pi/3)  SaturateOnIntegerOverflow=on  OutDataTypeStr=Inherit: Same as input  ParamDataTypeStr=Inherit: Same as input
  "a^2 " : Gain  Gain=exp(-j*2*pi/3)  SaturateOnIntegerOverflow=on  OutDataTypeStr=Inherit: Same as input  ParamDataTypeStr=Inherit: Same as input
  a^3 : Gain  Gain=1/3  SaturateOnIntegerOverflow=on  OutDataTypeStr=Inherit: Same as input  ParamDataTypeStr=Inherit: Same as input
  a^4 : Gain  Gain=2/3  SaturateOnIntegerOverflow=on  OutDataTypeStr=Inherit: Same as input  ParamDataTypeStr=Inherit: Same as input
  A : PMIOPort  Tag=PMCPort  Side=Left
  B : PMIOPort  Tag=PMCPort  Port=2  Side=Left
  C : PMIOPort  Tag=PMCPort  Port=3  Side=Left
  wires:
  Break Alg. Loop 1/1(Out) -> a^2/1, [Ia]
  Conj1/1 -> Break Alg. Loop 1/1(In)
  Avoid division by zero/1(O) -> Product/1  "V1"
  Load/1(PQ) -> Demux/1
  Demux/2 -> Real-Imag to Complex/2
  Demux/1 -> Real-Imag to Complex/1
  a^4/1 -> Conj1/1
  "a^2 "/1 -> Add/2
  [Vbc] -> "a^2 "/1
  [Vab] -> Add/1
  Add/1 -> a^3/1
  a^3/1 -> Avoid division by zero/1(I)
  a^2/1 -> [Ib]
  Product/1 -> a^4/1  "I1"
  Real-Imag to Complex/1 -> Product/2
  [Ib] -> CSb/1
  [Ia] -> Csa/1
  Voltage Measurement2/1 -> [Vbc]
  Voltage Measurement1/1 -> [Vab]
  connections:
  Series RLC Branch/RConn1 -- Series RLC Branch1/LConn1 -- B/RConn1 -- Voltage Measurement1/LConn2 -- Voltage Measurement2/LConn1 -- CSb/RConn1
  CSb/LConn1 -- Csa/LConn1 -- Series RLC Branch1/RConn1 -- C/RConn1 -- Voltage Measurement2/LConn2
  Voltage Measurement1/LConn1 -- Csa/RConn1 -- A/RConn1 -- Series RLC Branch/LConn1

== system ZEH_PV_grid/L11 ==
  note: V1= 1/3(Vab -a^2*Vbc)
  note: S = 3* ( V * I') / 2
  note: Ia= I1
  note: Ib= a^2*I1
  Add : Sum  Inputs=+-
  Avoid division by zero : Subsystem
  Break Alg. Loop 1 : Subsystem
  CSb : powerlib/Electrical Sources/Controlled Current Source  Initialize=on  Source_Type=AC  Amplitude=9355.5  Phase=(2.751-2*pi/3)*180/pi  Frequency=60  Measurements=Current
  Conj1 : Math  Operator=conj  SignedPower=on  SaturateOnIntegerOverflow=on
  Csa : powerlib/Electrical Sources/Controlled Current Source  Initialize=on  Source_Type=AC  Amplitude=9355.5  Phase=2.751*180/pi  Frequency=60  Measurements=Current
  Demux : Demux  Outputs=2
  Load : Subsystem
  Product : Product  Inputs=/*  InputSameDT=on  SaturateOnIntegerOverflow=on  OutDataTypeStr=Inherit: Same as first input
  Real-Imag to Complex : RealImagToComplex
  Series RLC Branch : powerlib/Elements/Series RLC Branch  LConnTagsString=__new0  RConnTagsString=__new0  BranchType=R  Resistance=1e6  Inductance=1e-3  SetiL0=off  InitialCurrent=0  Capacitance=1e-6  Setx0=off  InitialVoltage=0  Measurements=None
  Series RLC Branch1 : powerlib/Elements/Series RLC Branch  LConnTagsString=__new0  RConnTagsString=__new0  BranchType=R  Resistance=1e6  Inductance=1e-3  SetiL0=off  InitialCurrent=0  Capacitance=1e-6  Setx0=off  InitialVoltage=0  Measurements=None
  Voltage Measurement1 : powerlib/Measurements/Voltage Measurement  PhasorSimulation=on  OutputType=Complex  PSBequivalent=0
  Voltage Measurement2 : powerlib/Measurements/Voltage Measurement  PhasorSimulation=on  OutputType=Complex  PSBequivalent=0
  a^2 : Gain  Gain=exp(-j*2*pi/3)  SaturateOnIntegerOverflow=on  OutDataTypeStr=Inherit: Same as input  ParamDataTypeStr=Inherit: Same as input
  "a^2 " : Gain  Gain=exp(-j*2*pi/3)  SaturateOnIntegerOverflow=on  OutDataTypeStr=Inherit: Same as input  ParamDataTypeStr=Inherit: Same as input
  a^3 : Gain  Gain=1/3  SaturateOnIntegerOverflow=on  OutDataTypeStr=Inherit: Same as input  ParamDataTypeStr=Inherit: Same as input
  a^4 : Gain  Gain=2/3  SaturateOnIntegerOverflow=on  OutDataTypeStr=Inherit: Same as input  ParamDataTypeStr=Inherit: Same as input
  A : PMIOPort  Tag=PMCPort  Side=Left
  B : PMIOPort  Tag=PMCPort  Port=2  Side=Left
  C : PMIOPort  Tag=PMCPort  Port=3  Side=Left
  wires:
  Voltage Measurement1/1 -> [Vab]
  Voltage Measurement2/1 -> [Vbc]
  [Ia] -> Csa/1
  [Ib] -> CSb/1
  Real-Imag to Complex/1 -> Product/2
  Product/1 -> a^4/1  "I1"
  a^2/1 -> [Ib]
  a^3/1 -> Avoid division by zero/1(I)
  Add/1 -> a^3/1
  [Vab] -> Add/1
  [Vbc] -> "a^2 "/1
  "a^2 "/1 -> Add/2
  a^4/1 -> Conj1/1
  Demux/1 -> Real-Imag to Complex/1
  Demux/2 -> Real-Imag to Complex/2
  Load/1(PQ) -> Demux/1
  Avoid division by zero/1(O) -> Product/1  "V1"
  Conj1/1 -> Break Alg. Loop 1/1(In)
  Break Alg. Loop 1/1(Out) -> [Ia], a^2/1
  connections:
  Series RLC Branch/LConn1 -- A/RConn1 -- Csa/RConn1 -- Voltage Measurement1/LConn1
  Voltage Measurement2/LConn2 -- C/RConn1 -- Series RLC Branch1/RConn1 -- Csa/LConn1 -- CSb/LConn1
  CSb/RConn1 -- Voltage Measurement2/LConn1 -- Voltage Measurement1/LConn2 -- B/RConn1 -- Series RLC Branch1/LConn1 -- Series RLC Branch/RConn1

== system ZEH_PV_grid/L2 ==
  note: Ib= a^2*I1
  note: Ia= I1
  note: S = 3* ( V * I') / 2
  note: V1= 1/3(Vab -a^2*Vbc)
  Add : Sum  Inputs=+-
  Avoid division by zero : Subsystem
  Break Alg. Loop 1 : Subsystem
  CSb : powerlib/Electrical Sources/Controlled Current Source  Initialize=on  Source_Type=AC  Amplitude=9355.5  Phase=(2.751-2*pi/3)*180/pi  Frequency=60  Measurements=Current
  Conj1 : Math  Operator=conj  SignedPower=on  SaturateOnIntegerOverflow=on
  Csa : powerlib/Electrical Sources/Controlled Current Source  Initialize=on  Source_Type=AC  Amplitude=9355.5  Phase=2.751*180/pi  Frequency=60  Measurements=Current
  Demux : Demux  Outputs=2
  Load : Subsystem
  Product : Product  Inputs=/*  InputSameDT=on  SaturateOnIntegerOverflow=on  OutDataTypeStr=Inherit: Same as first input
  Real-Imag to Complex : RealImagToComplex
  Series RLC Branch : powerlib/Elements/Series RLC Branch  LConnTagsString=__new0  RConnTagsString=__new0  BranchType=R  Resistance=1e6  Inductance=1e-3  SetiL0=off  InitialCurrent=0  Capacitance=1e-6  Setx0=off  InitialVoltage=0  Measurements=None
  Series RLC Branch1 : powerlib/Elements/Series RLC Branch  LConnTagsString=__new0  RConnTagsString=__new0  BranchType=R  Resistance=1e6  Inductance=1e-3  SetiL0=off  InitialCurrent=0  Capacitance=1e-6  Setx0=off  InitialVoltage=0  Measurements=None
  Voltage Measurement1 : powerlib/Measurements/Voltage Measurement  PhasorSimulation=on  OutputType=Complex  PSBequivalent=0
  Voltage Measurement2 : powerlib/Measurements/Voltage Measurement  PhasorSimulation=on  OutputType=Complex  PSBequivalent=0
  a^2 : Gain  Gain=exp(-j*2*pi/3)  SaturateOnIntegerOverflow=on  OutDataTypeStr=Inherit: Same as input  ParamDataTypeStr=Inherit: Same as input
  "a^2 " : Gain  Gain=exp(-j*2*pi/3)  SaturateOnIntegerOverflow=on  OutDataTypeStr=Inherit: Same as input  ParamDataTypeStr=Inherit: Same as input
  a^3 : Gain  Gain=1/3  SaturateOnIntegerOverflow=on  OutDataTypeStr=Inherit: Same as input  ParamDataTypeStr=Inherit: Same as input
  a^4 : Gain  Gain=2/3  SaturateOnIntegerOverflow=on  OutDataTypeStr=Inherit: Same as input  ParamDataTypeStr=Inherit: Same as input
  A : PMIOPort  Tag=PMCPort  Side=Left
  B : PMIOPort  Tag=PMCPort  Port=2  Side=Left
  C : PMIOPort  Tag=PMCPort  Port=3  Side=Left
  wires:
  Break Alg. Loop 1/1(Out) -> a^2/1, [Ia]
  Conj1/1 -> Break Alg. Loop 1/1(In)
  Avoid division by zero/1(O) -> Product/1  "V1"
  Load/1(PQ) -> Demux/1
  Demux/2 -> Real-Imag to Complex/2
  Demux/1 -> Real-Imag to Complex/1
  a^4/1 -> Conj1/1
  "a^2 "/1 -> Add/2
  [Vbc] -> "a^2 "/1
  [Vab] -> Add/1
  Add/1 -> a^3/1
  a^3/1 -> Avoid division by zero/1(I)
  a^2/1 -> [Ib]
  Product/1 -> a^4/1  "I1"
  Real-Imag to Complex/1 -> Product/2
  [Ib] -> CSb/1
  [Ia] -> Csa/1
  Voltage Measurement2/1 -> [Vbc]
  Voltage Measurement1/1 -> [Vab]
  connections:
  Series RLC Branch/RConn1 -- Series RLC Branch1/LConn1 -- B/RConn1 -- Voltage Measurement1/LConn2 -- Voltage Measurement2/LConn1 -- CSb/RConn1
  CSb/LConn1 -- Csa/LConn1 -- Series RLC Branch1/RConn1 -- C/RConn1 -- Voltage Measurement2/LConn2
  Voltage Measurement1/LConn1 -- Csa/RConn1 -- A/RConn1 -- Series RLC Branch/LConn1

== system ZEH_PV_grid/L3 ==
  note: V1= 1/3(Vab -a^2*Vbc)
  note: S = 3* ( V * I') / 2
  note: Ia= I1
  note: Ib= a^2*I1
  Add : Sum  Inputs=+-
  Avoid division by zero : Subsystem
  Break Alg. Loop 1 : Subsystem
  CSb : powerlib/Electrical Sources/Controlled Current Source  Initialize=on  Source_Type=AC  Amplitude=9355.5  Phase=(2.751-2*pi/3)*180/pi  Frequency=60  Measurements=Current
  Conj1 : Math  Operator=conj  SignedPower=on  SaturateOnIntegerOverflow=on
  Csa : powerlib/Electrical Sources/Controlled Current Source  Initialize=on  Source_Type=AC  Amplitude=9355.5  Phase=2.751*180/pi  Frequency=60  Measurements=Current
  Demux : Demux  Outputs=2
  Load : Subsystem
  Product : Product  Inputs=/*  InputSameDT=on  SaturateOnIntegerOverflow=on  OutDataTypeStr=Inherit: Same as first input
  Real-Imag to Complex : RealImagToComplex
  Series RLC Branch : powerlib/Elements/Series RLC Branch  LConnTagsString=__new0  RConnTagsString=__new0  BranchType=R  Resistance=1e6  Inductance=1e-3  SetiL0=off  InitialCurrent=0  Capacitance=1e-6  Setx0=off  InitialVoltage=0  Measurements=None
  Series RLC Branch1 : powerlib/Elements/Series RLC Branch  LConnTagsString=__new0  RConnTagsString=__new0  BranchType=R  Resistance=1e6  Inductance=1e-3  SetiL0=off  InitialCurrent=0  Capacitance=1e-6  Setx0=off  InitialVoltage=0  Measurements=None
  Voltage Measurement1 : powerlib/Measurements/Voltage Measurement  PhasorSimulation=on  OutputType=Complex  PSBequivalent=0
  Voltage Measurement2 : powerlib/Measurements/Voltage Measurement  PhasorSimulation=on  OutputType=Complex  PSBequivalent=0
  a^2 : Gain  Gain=exp(-j*2*pi/3)  SaturateOnIntegerOverflow=on  OutDataTypeStr=Inherit: Same as input  ParamDataTypeStr=Inherit: Same as input
  "a^2 " : Gain  Gain=exp(-j*2*pi/3)  SaturateOnIntegerOverflow=on  OutDataTypeStr=Inherit: Same as input  ParamDataTypeStr=Inherit: Same as input
  a^3 : Gain  Gain=1/3  SaturateOnIntegerOverflow=on  OutDataTypeStr=Inherit: Same as input  ParamDataTypeStr=Inherit: Same as input
  a^4 : Gain  Gain=2/3  SaturateOnIntegerOverflow=on  OutDataTypeStr=Inherit: Same as input  ParamDataTypeStr=Inherit: Same as input
  A : PMIOPort  Tag=PMCPort  Side=Left
  B : PMIOPort  Tag=PMCPort  Port=2  Side=Left
  C : PMIOPort  Tag=PMCPort  Port=3  Side=Left
  wires:
  Voltage Measurement1/1 -> [Vab]
  Voltage Measurement2/1 -> [Vbc]
  [Ia] -> Csa/1
  [Ib] -> CSb/1
  Real-Imag to Complex/1 -> Product/2
  Product/1 -> a^4/1  "I1"
  a^2/1 -> [Ib]
  a^3/1 -> Avoid division by zero/1(I)
  Add/1 -> a^3/1
  [Vab] -> Add/1
  [Vbc] -> "a^2 "/1
  "a^2 "/1 -> Add/2
  a^4/1 -> Conj1/1
  Demux/1 -> Real-Imag to Complex/1
  Demux/2 -> Real-Imag to Complex/2
  Load/1(PQ) -> Demux/1
  Avoid division by zero/1(O) -> Product/1  "V1"
  Conj1/1 -> Break Alg. Loop 1/1(In)
  Break Alg. Loop 1/1(Out) -> [Ia], a^2/1
  connections:
  Series RLC Branch/LConn1 -- A/RConn1 -- Csa/RConn1 -- Voltage Measurement1/LConn1
  Voltage Measurement2/LConn2 -- C/RConn1 -- Series RLC Branch1/RConn1 -- Csa/LConn1 -- CSb/LConn1
  CSb/RConn1 -- Voltage Measurement2/LConn1 -- Voltage Measurement1/LConn2 -- B/RConn1 -- Series RLC Branch1/LConn1 -- Series RLC Branch/RConn1
